simulink model "rst"  (R2023b)
settings: Solver=VariableStepAuto  StartTime=0.0  StopTime=60.0  RelTol=1e-3
settings Model: Creator=kamic  LastModifiedBy=kamic

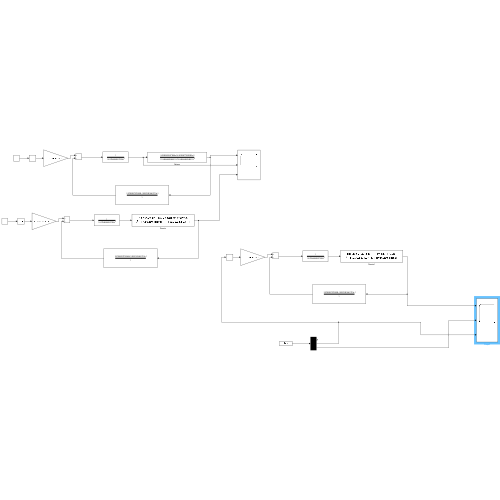
[thumbnail: Simulink's stored preview of the top-level diagram]
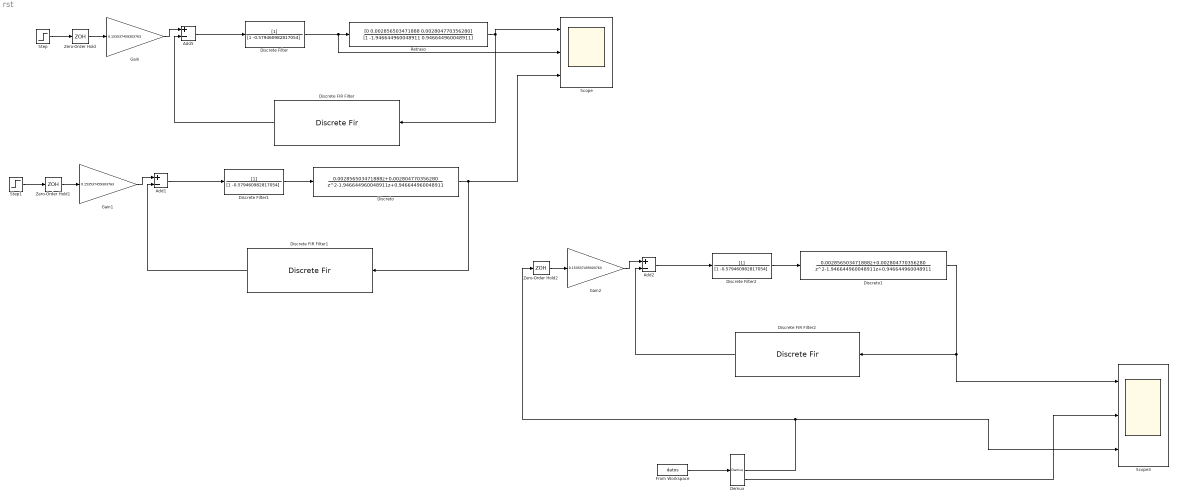
== system rst ==
  Add1 : Sum  Inputs=+-
  Add2 : Sum  Inputs=+-
  Add5 : Sum  Inputs=+-
  Demux : Demux  Outputs=3
  Discrete FIR Filter : DiscreteFir  Coefficients=[ 2.079050275705499 -1.925512816401701]
  Discrete FIR Filter1 : DiscreteFir  Coefficients=[ 2.079050275705499 -1.925512816401701]
  Discrete FIR Filter2 : DiscreteFir  Coefficients=[ 2.079050275705499 -1.925512816401701]
  Discrete Filter : DiscreteFilter  Denominator=[1 -0.579460982817054]
  Discrete Filter1 : DiscreteFilter  Denominator=[1 -0.579460982817054]
  Discrete Filter2 : DiscreteFilter  Denominator=[1 -0.579460982817054]
  Discreto : DiscreteTransferFcn  Numerator=[0 0.002856503471888 0.002804770356280]  Denominator=[1 -1.946644960048911 0.946644960048911]
  Discreto1 : DiscreteTransferFcn  Numerator=[0 0.002856503471888 0.002804770356280]  Denominator=[1 -1.946644960048911 0.946644960048911]
  From Workspace : FromWorkspace  VariableName=datos  SampleTime=0.01
  Gain : Gain  Gain=0.153537459303763
  Gain1 : Gain  Gain=0.153537459303763
  Gain2 : Gain  Gain=0.153537459303763
  Retraso : DiscreteFilter  Numerator=[0 0.002856503471888 0.002804770356280]  Denominator=[1 -1.946644960048911 0.946644960048911]
  Scope : Scope  NumInputPorts=3
  Scope3 : Scope  NumInputPorts=3
  Step : Step  Time=0  SampleTime=0
  Step1 : Step  Time=0  SampleTime=0
  Zero-Order Hold : ZeroOrderHold  SampleTime=0.01
  Zero-Order Hold1 : ZeroOrderHold  SampleTime=0.01
  Zero-Order Hold2 : ZeroOrderHold  SampleTime=0.01
  wires:
  Step/1 -> Zero-Order Hold/1
  Gain/1 -> Add5/1
  Discrete Filter/1 -> Retraso/1, Scope/2
  Add5/1 -> Discrete Filter/1
  Retraso/1 -> Discrete FIR Filter/1, Scope/1
  Discrete FIR Filter/1 -> Add5/2
  Zero-Order Hold/1 -> Gain/1
  Add1/1 -> Discrete Filter1/1
  Step1/1 -> Zero-Order Hold1/1
  Discrete Filter1/1 -> Discreto/1
  Discreto/1 -> Scope/3, Discrete FIR Filter1/1
  Discrete FIR Filter1/1 -> Add1/2
  Zero-Order Hold1/1 -> Gain1/1
  Gain1/1 -> Add1/1
  Gain2/1 -> Add2/1
  Discreto1/1 -> Scope3/1, Discrete FIR Filter2/1
  Discrete Filter2/1 -> Discreto1/1
  Zero-Order Hold2/1 -> Gain2/1
  Demux/2 -> Zero-Order Hold2/1, Scope3/3
  From Workspace/1 -> Demux/1
  Demux/3 -> Scope3/2
  Add2/1 -> Discrete Filter2/1
  Discrete FIR Filter2/1 -> Add2/2
